simulink model "Parking_NMPC_Controller"  (R2024b)
settings: configuration reference "vehicle_nl_controller_config" (kept outside this file)
undefined symbols (not defined in the file or in its folder): refNum, TimeStep, u0, wheel_base
libraries: mpclib x1, nl_vehicle_MPC_lib x1
settings Model: DataDictionary=sim_data_vehicle_nl.sldd  Creator=tshintai  LastModifiedBy=tshintai
settings ConfigSetRef: SourceName=vehicle_nl_controller_config

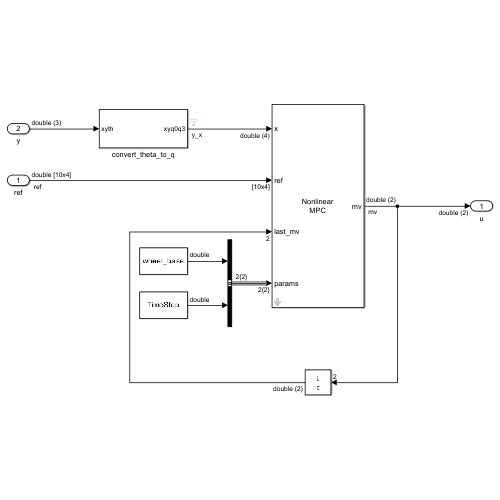
[thumbnail: Simulink's stored preview of the top-level diagram]
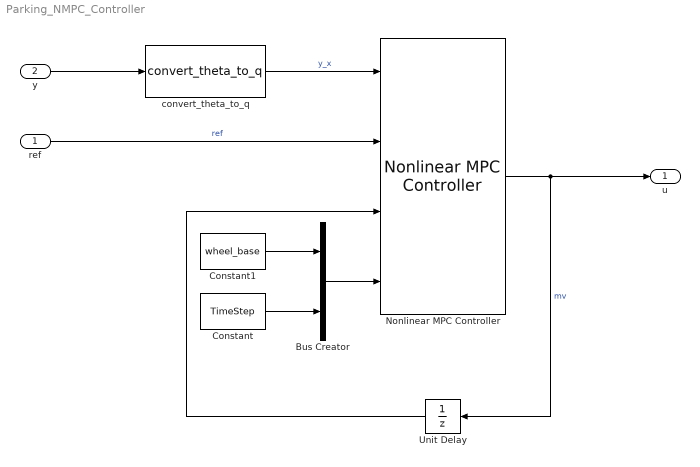
== system Parking_NMPC_Controller ==
  ref : Inport  OutDataTypeStr=double  PortDimensions=[refNum, 4]
  y : Inport  Port=2  OutDataTypeStr=double  PortDimensions=3
  Bus Creator : BusCreator  Inputs=2  OutDataTypeStr=Bus: NLMPC_param_bus
      settings: InheritFromInputs=off
  Constant : Constant  Value=TimeStep
  Constant1 : Constant  Value=wheel_base
  Nonlinear MPC Controller : mpclib/Nonlinear MPC Controller  SCDEnableBlockLinearizationSpecification=on  nlmpcobj=nlMPCObj  UseObjectTs=on  UseMEX=off  mexname='nlMPCObj_mex'  md_enabled=off  mvtarget_enabled=off  param_enabled=on  cost_enabled=off  mvseq_enabled=off  stateseq_enabled=off  ovseq_enabled=off  slack_enabled=off  status_enabled=off  ov_min=off  ov_max=off  mv_min=off  mv_max=off  mvrate_min=off  mvrate_max=off  state_min=off  state_max=off  ov_weight=off  mv_weight=off  mvrate_weight=off  ecr_weight=off  nlp_initialize=off
  Unit Delay : UnitDelay  InitialCondition=u0  SampleTime=-1  HasFrameUpgradeWarning=on
  convert_theta_to_q : nl_vehicle_MPC_lib/convert_theta_to_q  SystemSampleTime=-1  VariantActivationTime=update diagram  AllowFlexibleInterface=on  Latency=0  AutoFrameSizeCalculation=off
  u : Outport  OutDataTypeStr=double  PortDimensions=2
  wires:
  Nonlinear MPC Controller/1 -> Unit Delay/1, u/1  "mv"
  Unit Delay/1 -> Nonlinear MPC Controller/3
  y/1 -> convert_theta_to_q/1
  Bus Creator/1 -> Nonlinear MPC Controller/4
  Constant/1 -> Bus Creator/2
  Constant1/1 -> Bus Creator/1
  convert_theta_to_q/1 -> Nonlinear MPC Controller/1  "y_x"
  ref/1 -> Nonlinear MPC Controller/2  "ref"
